simulink model "SDV_HIL"  (R2025a)
settings: Solver=VariableStepAuto  StartTime=0.0  StopTime=9999  FixedStep=0.001  RelTol=1e-3
undefined symbols (not defined in the file): Breakpoints_Fz, Cij, dspblkCoreblockFVToolHelper, eta, Fx_total_max, g, gcbh, Iz, lambda, lf, lr, mu, phi, R_eff, Tmax, xi
libraries: simulink_extras x30, slrealtimeiplib x17, slpidlib x16, simulink x10, SignalEditorBlockLib x6, dspstat3 x5, Solver_SF x3, sl3dlib x3
(part 2 of 5)

== system SDV_HIL/HIL_VCU/UDP Receive ZCU -> PC ==
  Display18 : Display
  Display26 : Display  Commented=on
  Gain1 : Gain  Gain=-1
  MATLAB Function : MATLAB Function  TreatAsAtomicUnit=on
  Median Filter : dspstat3/Median Filter  Commented=on  WindowLength=5  SimulateUsing=Interpreted execution
      settings: LibrarySourceBlock=|
      | dspfdesign/Median
      | Filter
  Mux : Mux
  Mux1 : Mux
  Rate Transition2 : RateTransition  OutPortSampleTime=0.0001
  Scope : Scope  Commented=on  NumInputPorts=2
      settings: TimeSpan=10  ActiveDisplayYMinimum=-148.76999999999998  ActiveDisplayYMaximum=138.92999999999998  DataLoggingVariableName=ScopeData62
  Scope1 : Scope  Commented=on
      settings: ActiveDisplayYMinimum=-50  ActiveDisplayYMaximum=-30  DataLoggingVariableName=ScopeData63
  Spd & Ang Convertion2 : Subsystem
  UDP Receive3 : slrealtimeiplib/UDP Receive  useHostTargetConn=off  ipAddress=10.252.62.212  localPort=4095  rcvWidth=7  rcvFmAny=on  fmAddress='10.252.62.51'  sampleTime=0.0001  enableMessage=off  maxPackets=1
  vxWheel_Ref : Outport
  AngWheel : Outport  Port=2
  wires:
  MATLAB Function/5(seqRecv) -> Display26/1
  UDP Receive3/2 -> Display18/1
  UDP Receive3/1 -> Rate Transition2/1
  Rate Transition2/1 -> MATLAB Function/1(payload)
  MATLAB Function/4(RR) -> Spd & Ang Convertion2/4(RR)
  MATLAB Function/3(RL) -> Spd & Ang Convertion2/3(RL)
  MATLAB Function/2(FR) -> Spd & Ang Convertion2/2(FR)
  MATLAB Function/1(FL) -> Spd & Ang Convertion2/1(FL)
  Spd & Ang Convertion2/1(ang_FL) -> Mux/1
  Spd & Ang Convertion2/2(ang_FR) -> Mux/2
  Spd & Ang Convertion2/3(ang_RL) -> Mux/3
  Spd & Ang Convertion2/4(ang_RR) -> Mux/4
  Mux/1 -> Gain1/1
  Spd & Ang Convertion2/5(vxWheel_FL) -> Mux1/1
  Spd & Ang Convertion2/6(vxWheel_FR) -> Mux1/2
  Spd & Ang Convertion2/7(vxWheel_RL) -> Mux1/3
  Spd & Ang Convertion2/8(vxWheel_RR) -> Mux1/4
  Median Filter/1 -> Scope/2
  Mux1/1 -> Median Filter/1, vxWheel_Ref/1, Scope/1
  Gain1/1 -> Scope1/1, AngWheel/1

== system SDV_HIL/HIL_VCU/UDP Receive Brake VCU -> PC ==
  Cast To Double : DataTypeConversion  OutDataTypeStr=double  SaturateOnIntegerOverflow=off  RndMeth=Floor
  Constant : Constant  Value=10
  Display : Display
  Display1 : Display
  Divide : Product  Inputs=*/
  MATLAB Function : MATLAB Function  TreatAsAtomicUnit=on
  Rate Transition : RateTransition  OutPortSampleTime=0.0001
  UDP Receive : slrealtimeiplib/UDP Receive  useHostTargetConn=off  ipAddress=10.252.62.212  localPort=4093  rcvWidth=4  rcvFmAny=on  fmAddress='10.10.10.10'  sampleTime=0.0001  enableMessage=off  maxPackets=1
  Brake : Outport
  wires:
  UDP Receive/2 -> Display/1
  MATLAB Function/2(seqRecv) -> Display1/1
  Constant/1 -> Divide/2
  MATLAB Function/1(Brake) -> Divide/1
  Divide/1 -> Cast To Double/1
  Cast To Double/1 -> Brake/1
  UDP Receive/1 -> Rate Transition/1
  Rate Transition/1 -> MATLAB Function/1(payload)

== system SDV_HIL/HIL_VCU/UDP Transmit PC -> VCU ==
  Vx : Inport
  Vy : Inport  Port=2
  AngWheel : Inport  Port=3
  r : Inport  Port=4
  Fy : Inport  Port=5
  Fz : Inport  Port=6
  VxWheel : Inport  Port=7
  Cast To Double : DataTypeConversion  OutDataTypeStr=double  SaturateOnIntegerOverflow=off  RndMeth=Floor
  Cast To Double1 : DataTypeConversion  OutDataTypeStr=double  SaturateOnIntegerOverflow=off  RndMeth=Floor
  Display{3..9} (7 alike) : Display
  MATLAB Function1 : MATLAB Function  TreatAsAtomicUnit=on
  UDP Send : slrealtimeiplib/UDP Send  useHostTargetConn=off  toAddress='10.252.62.129'  toPort=5100  sampleTime=0.001  enableMessage=off  ipAddress=10.252.62.212  localPort=4095
  UDP Send5 : slrealtimeiplib/UDP Send  useHostTargetConn=off  toAddress='10.252.62.55'  toPort=5055  sampleTime=0.001  enableMessage=off  ipAddress=10.252.62.212  localPort=4095
  wires:
  r/1 -> Display5/1, MATLAB Function1/4(r)
  Vy/1 -> Display3/1, MATLAB Function1/2(Vy)
  MATLAB Function1/1(payload) -> UDP Send/1, UDP Send5/1
  VxWheel/1 -> Display6/1, MATLAB Function1/7(Vx_wheel)
  AngWheel/1 -> Display4/1, MATLAB Function1/3(AngWheel)
  Fy/1 -> Display8/1, MATLAB Function1/5(Fy)
  Fz/1 -> Display9/1, MATLAB Function1/6(Fz)
  Vx/1 -> Display7/1, MATLAB Function1/1(Vx)
  MATLAB Function1/2(len) -> Cast To Double1/1, Cast To Double/1
  Cast To Double/1 -> UDP Send5/2
  Cast To Double1/1 -> UDP Send/2

== system SDV_HIL/Draft1/Sensor1/Steering System ==
  In1 : Inport
  Demux : Demux  Outputs=14
  Terminator{,1..7} (8 alike) : Terminator
  tag scope: Lat_Path=global, Lat_Targ=global, Lat_Veh=global, SteerDM=global, sideslip_L2=global, sideslip_R2=global
  wires:
  In1/1 -> Demux/1
  Demux/1 -> Terminator/1
  Demux/2 -> Terminator1/1
  Demux/3 -> Terminator2/1
  Demux/4 -> Terminator3/1
  Demux/5 -> Terminator4/1
  Demux/6 -> Terminator5/1
  Demux/7 -> [SteerDM]
  Demux/8 -> [Lat_Targ]
  Demux/9 -> [Lat_Veh]
  Demux/10 -> [Lat_Path]
  Demux/11 -> Terminator6/1
  Demux/12 -> Terminator7/1
  Demux/13 -> [sideslip_L2]
  Demux/14 -> [sideslip_R2]

== system SDV_HIL/Draft1/Sensor1/Torque Vectoring ==
  In1 : Inport
  Degrees to Radians : simulink_extras/Transformations/Degrees to Radians
  Degrees to Radians2 : simulink_extras/Transformations/Degrees to Radians
  Demux : Demux  Outputs=15
  Mux : Mux
  Mux1 : Mux
  Mux2 : Mux
  Scope{,2..5} (5 alike) : Scope  Commented=on
      Scope settings: TimeSpan=10  ActiveDisplayYMinimum=-0.018082463921750395  ActiveDisplayYMaximum=0.017846570793703453  DataLoggingVariableName=ScopeData21
      Scope2 settings: ActiveDisplayYMinimum=-1  ActiveDisplayYMaximum=1  DataLoggingVariableName=ScopeData23
      Scope3 settings: ActiveDisplayYMinimum=-106.0637202101492  ActiveDisplayYMaximum=78.0503751303972  DataLoggingVariableName=ScopeData24
      Scope4 settings: ActiveDisplayYMinimum=6542.1615610939225  ActiveDisplayYMaximum=6577.8874866083952  DataLoggingVariableName=ScopeData25
      Scope5 settings: TimeSpan=10  ActiveDisplayYMinimum=-11.664536557177181  ActiveDisplayYMaximum=101.92313834201745  DataLoggingVariableName=ScopeData61
  Scope1 : Scope  Commented=on  NumInputPorts=2
      settings: ActiveDisplayYMinimum=-15.76512014934719  ActiveDisplayYMaximum=98.336342875694754  DataLoggingVariableName=ScopeData22
  tag scope: AngWheel=global, Fy=global, Fz=global, Vx=global, Vy=global, yawrate=global
  wires:
  In1/1 -> Demux/1
  Demux/1 -> Scope5/1, [Vx]
  Demux/2 -> Scope2/1, [Vy]
  Demux/3 -> Degrees to Radians/1
  Demux/4 -> Mux2/1
  Demux/5 -> Mux2/2
  Demux/6 -> Mux2/3
  Demux/7 -> Mux2/4
  Demux/8 -> Mux1/1
  Demux/9 -> Mux1/2
  Demux/10 -> Mux1/3
  Demux/11 -> Mux1/4
  Demux/12 -> Mux/1
  Demux/13 -> Mux/2
  Demux/14 -> Mux/3
  Demux/15 -> Mux/4
  Degrees to Radians/1 -> Scope/1, [yawrate]
  Mux/1 -> Scope3/1, [Fy]
  Mux1/1 -> Scope4/1, [Fz]
  Mux2/1 -> Scope1/2, Degrees to Radians2/1
  Degrees to Radians2/1 -> Scope1/1, [AngWheel]

== system SDV_HIL/Draft1/Sensor1/Traction Control ==
  In1 : Inport
  Demux : Demux  Outputs=14
  Gain{,1..3} (4 alike) : Gain  Gain=2*pi/60
  Mux : Mux
  Mux1 : Mux
  Terminator : Terminator
  g > m/s^2 : Gain  Gain=9.80665
  tag scope: Fx=global, VxWheel=global, Vx_L1=global, Vx_L2=global, Vx_R1=global, Vx_R2=global, ax=global, w_L1=global, w_L2=global, w_R1=global, w_R2=global
  wires:
  In1/1 -> Demux/1
  Demux/2 -> [Vx_L1]
  Demux/3 -> [Vx_R1]
  Demux/4 -> [Vx_L2]
  Demux/5 -> [Vx_R2]
  Demux/1 -> Terminator/1  "Vx"
  Demux/6 -> Gain/1
  Demux/7 -> Gain1/1
  Demux/8 -> Gain2/1
  Demux/9 -> Gain3/1
  Gain/1 -> [w_L1]
  Gain1/1 -> [w_R1]
  Gain2/1 -> [w_L2]
  Gain3/1 -> [w_R2]
  Demux/10 -> g > m/s^2/1
  g > m/s^2/1 -> [ax]
  Demux/14 -> Mux/4  "Fx_R2"
  Demux/13 -> Mux/3  "Fx_L2"
  Demux/12 -> Mux/2  "Fx_R1"
  Demux/11 -> Mux/1  "Fx_L1"
  Mux/1 -> [Fx]
  [Vx_L1] -> Mux1/1
  [Vx_R1] -> Mux1/2
  [Vx_L2] -> Mux1/3
  [Vx_R2] -> Mux1/4
  Mux1/1 -> [VxWheel]

== system SDV_HIL/Draft1/Steering Input1/DLC Lateral Target  ==
  PID Controller : slpidlib/PID Controller  Controller=PID  Form=Parallel  TimeDomain=Continuous-time  UseExternalTs=off  SampleTime=-1  IntegratorMethod=Forward Euler  FilterMethod=Forward Euler  ControllerParametersSource=internal  P=12  I=0.7  UseKiTs=off  D=7  UseExternalDerivativeSource=off  N=100  UseFilter=on  TunerSelectOption=Transfer Function Based (PID Tuner App)  InitialConditionSource=internal  InitialConditionForIntegrator=0  InitialConditionForFilter=0  DifferentiatorICPrevScaledInput=0  ExternalReset=none  TrackingMode=off  Kt=1  LimitOutput=off  SatLimitsSource=internal  UpperSaturationLimit=inf  LowerSaturationLimit=-inf  LinearizeAsGain=on  AntiWindupMode=none  Kb=1  LimitIntegrator=off  UpperIntegratorSaturationLimit=inf  LowerIntegratorSaturationLimit=-inf  POutMin=[]  POutMax=[]  IOutMin=[]  IOutMax=[]  DOutMin=[]  DOutMax=[]  NOutMin=[]  NOutMax=[]  SumOutMin=[]  SumOutMax=[]  SaturationOutMin=[]  SaturationOutMax=[]  PParamMin=[]  PParamMax=[]  IParamMin=[]  IParamMax=[]  DParamMin=[]  DParamMax=[]  NParamMin=[]  NParamMax=[]  KbParamMin=[]  KbParamMax=[]  KtParamMin=[]  KtParamMax=[]  KbOutMin=[]  KbOutMax=[]  KtOutMin=[]  KtOutMax=[]  IntegratorOutMin=[]  IntegratorOutMax=[]  FilterOutMin=[]  FilterOutMax=[]  SumI1OutMin=[]  SumI1OutMax=[]  SumI2OutMin=[]  SumI2OutMax=[]  SumI3OutMin=[]  SumI3OutMax=[]  SumI4OutMin=[]  SumI4OutMax=[]  SumDOutMin=[]  SumDOutMax=[]  DifferentiatorOutMin=[]  DifferentiatorOutMax=[]  FilterDiffOutCoefMin=[]  FilterDiffOutCoefMax=[]  ReciprocalOutMin=[]  ReciprocalOutMax=[]  SumDenOutMin=[]  SumDenOutMax=[]  SumNumOutMin=[]  SumNumOutMax=[]  DivideOutMin=[]  DivideOutMax=[]  UdiffTsProdOutMin=[]  UdiffTsProdOutMax=[]  NTsProdOutMin=[]  NTsProdOutMax=[]  UintegralTsProdOutMin=[]  UintegralTsProdOutMax=[]  UngainTsProdOutMin=[]  UngainTsProdOutMax=[]  ClampingZeroOutDataTypeStr=Inherit: Inherit via back propagation  ClampingZeroOutMin=[]  ClampingZeroOutMax=[]  FilterDenConstantOutDataTypeStr=Inherit: Inherit via back propagation  FilterDenConstantOutMin=[]  FilterDenConstantOutMax=[]  PCopyOutDataTypeStr=Inherit: Inherit via back propagation  PCopyOutMin=[]  PCopyOutMax=[]  NCopyOutDataTypeStr=Inherit: Inherit via back propagation  NCopyOutMin=[]  NCopyOutMax=[]  IntegratorContinuousStateAttributes=''  IntegratorStateMustResolveToSignalObject=off  IntegratorRTWStateStorageClass=Auto  FilterContinuousStateAttributes=''  FilterStateMustResolveToSignalObject=off  FilterRTWStateStorageClass=Auto  ParallelPVariant=InternalParameters  IdealPVariant=Disabled  IVariant=InternalParameters  DVariant=InternalParameters  IntegratorVariant=Continuous  SatVariant=Disabled  AWVariant=Passthrough  PCopyVariant=Disabled  TRVariant=Disabled  FdbkBlocksVariant=Forward  IdealPFdbkVariant=Disabled  SatFdbkVariant=Disabled  DerivativeFilterVariant=ContFilter  NVariant=InternalParameters  NCopyVariant=Disabled  FilterICVariant=InternalICsFilter  IntegratorICVariant=InternalICs  ExternalResetVariant=Disabled  TRSumVariant=Passthrough  SumFdbkVariant=Disabled  SumVariant=Sum_PID  TsampFilterVariant=InternalTs  TsampNgainVariant=Passthrough  TsampIntegralVariant=Disabled_SignalSpec  ExternalSaturationOutDataTypeStr=Inherit: Same as second input  DerivativeSourceVariant=ErrorSignal  PreIntVariant=InternalPreInt
  Saturation : Saturate  UpperLimit=40  LowerLimit=-40
  Scope1 : Scope
      settings: ActiveDisplayYMinimum=-50  ActiveDisplayYMaximum=50  DataLoggingVariableName=ScopeData17
  Scope2 : Scope
      settings: ActiveDisplayYMinimum=-26.333159271082913  ActiveDisplayYMaximum=27.304615856489622  DataLoggingVariableName=ScopeData18
  Sum : Sum  Inputs=|+-
  Out1 : Outport
  wires:
  [Lat_Veh] -> Sum/2
  [Lat_Targ] -> Sum/1
  Sum/1 -> Scope2/1, PID Controller/1
  PID Controller/1 -> Saturation/1
  Saturation/1 -> Out1/1, Scope1/1

== system SDV_HIL/Draft1/Steering Input1/DLC SteerDM ==
  1-D Lookup Table : Lookup_n-D  NumberOfTableDimensions=1  BreakpointsForDimension1=[-540 0 540]  Table=[-40 0 40]  InternalRulePriority=Speed  RndMeth=Simplest
  Saturation : Saturate  UpperLimit=40  LowerLimit=-40
  Scope1 : Scope  NumInputPorts=3
      settings: ActiveDisplayYMinimum=-1  ActiveDisplayYMaximum=1  DataLoggingVariableName=ScopeData19
  Str : Outport
  wires:
  Saturation/1 -> Str/1, Scope1/1
  1-D Lookup Table/1 -> Scope1/2, Saturation/1
  [SteerDM] -> 1-D Lookup Table/1, Scope1/3

== system SDV_HIL/Draft1/Steering Input1/Driver Logi G29 ==
  Add : Sum
  Add1 : Sum
  Constant : Constant  Value=50
  Constant1 : Constant  Value=6
  Demux : Demux
  Display{,1..2,4..6} (6 alike) : Display
  Gain3 : Gain  Gain=-6
  Gain4 : Gain  Gain=-50
  Gain5 : Gain  Gain=40
  Goto2 : Goto  Commented=on  GotoTag=Brake_pedal  TagVisibility=global
  MATLAB Function : MATLAB Function  TreatAsAtomicUnit=on
  Selector : Selector  InputPortWidth=25  IndexOptions=Index vector (dialog)  Indices=[1]  OutputSizes=1
  Simulation 3D Joystick : sl3dlib/Simulation 3D/Hardware Interface/Simulation 3D Joystick  joyid=1  adjustports=on  forcefeed=off
  Switch : Switch  Criteria=u2 > Threshold  SaturateOnIntegerOverflow=off  InputSameDT=off
  Switch1 : Switch  Criteria=u2 > Threshold  SaturateOnIntegerOverflow=off  InputSameDT=off
  Terminator : Terminator
  Terminator2 : Terminator
  Zero : Constant  Value=0  OutDataTypeStr=Inherit: Inherit via back propagation
  Zero1 : Constant  Value=0  OutDataTypeStr=Inherit: Inherit via back propagation
  tag scope: Steer=global, Throttle=global
  wires:
  Simulation 3D Joystick/3 -> Terminator/1
  Zero1/1 -> Switch1/3
  Switch1/1 -> Display5/1, [Throttle]
  Add/1 -> Switch1/1
  Zero/1 -> Switch/3
  MATLAB Function/1(state) -> Display4/1, Switch/2, Switch1/2
  Selector/1 -> MATLAB Function/1(btn)
  Gain5/1 -> [Steer], Display2/1
  Add1/1 -> Display6/1, Goto2/1
  Constant1/1 -> Add1/2
  Gain3/1 -> Add1/1
  Demux/3 -> Gain3/1
  Demux/2 -> Gain4/1
  Demux/1 -> Gain5/1
  Demux/4 -> Terminator2/1
  Simulation 3D Joystick/1 -> Display/1, Demux/1, Switch/1
  Gain4/1 -> Add/1
  Constant/1 -> Add/2
  Simulation 3D Joystick/2 -> Selector/1, Display1/1

== system SDV_HIL/Draft1/Steering Input1/Sine with Dwell ==
  Gain : Gain  Gain=5
  Sine with Dwell : SignalEditorBlockLib/Signal Editor  FileName=Sine with Dwell.mat  ActiveScenario=Scenario  ActiveSignal=Signal 1  IsBus=off  OutputBusObjectStr=Bus: BusObject  SampleTime=0  ZeroCross=off  OutputAfterFinalValue=Setting to zero  Unit=inherit  PreserveSignalName=on  ApplySigPropsToAllScenarios=on  ApplySigPropsToAllSignals=off  SignalPropertySource=Dialog parameters
  Str : Outport
  wires:
  Sine with Dwell/1 -> Gain/1
  Gain/1 -> Str/1

== system SDV_HIL/Draft1/Steering Input1/Sine with Dwell shifted ==
  Gain : Gain  Gain=5
  Sine with Dwell : SignalEditorBlockLib/Signal Editor  FileName=SineWithDwell_shifted.mat  ActiveScenario=Scenario  ActiveSignal=Signal 1  IsBus=off  OutputBusObjectStr=Bus: BusObject  SampleTime=0  ZeroCross=off  OutputAfterFinalValue=Setting to zero  Unit=inherit  PreserveSignalName=on  ApplySigPropsToAllScenarios=on  ApplySigPropsToAllSignals=off  SignalPropertySource=Dialog parameters
  Str : Outport
  wires:
  Gain/1 -> Str/1
  Sine with Dwell/1 -> Gain/1

== system SDV_HIL/Draft1/Steering Input1/Subsystem ==
  In1 : Inport
  Str : Outport
  wires:
  In1/1 -> Str/1

== system SDV_HIL/Draft1/Subsystem1/Motor1 ==
  SpdTCS : Inport
  Demux : Demux
  Gain : Gain  Gain=4
  Mux : Mux
  PID Controller : slpidlib/PID Controller  Controller=PID  Form=Parallel  TimeDomain=Continuous-time  UseExternalTs=off  SampleTime=-1  IntegratorMethod=Forward Euler  FilterMethod=Forward Euler  ControllerParametersSource=internal  P=20  I=0.05  UseKiTs=off  D=1  UseExternalDerivativeSource=off  N=100  UseFilter=on  TunerSelectOption=Transfer Function Based (PID Tuner App)  InitialConditionSource=internal  InitialConditionForIntegrator=0  InitialConditionForFilter=0  DifferentiatorICPrevScaledInput=0  ExternalReset=none  TrackingMode=off  Kt=1  LimitOutput=off  SatLimitsSource=internal  UpperSaturationLimit=inf  LowerSaturationLimit=-inf  LinearizeAsGain=on  AntiWindupMode=none  Kb=1  LimitIntegrator=off  UpperIntegratorSaturationLimit=inf  LowerIntegratorSaturationLimit=-inf  POutMin=[]  POutMax=[]  IOutMin=[]  IOutMax=[]  DOutMin=[]  DOutMax=[]  NOutMin=[]  NOutMax=[]  SumOutMin=[]  SumOutMax=[]  SaturationOutMin=[]  SaturationOutMax=[]  PParamMin=[]  PParamMax=[]  IParamMin=[]  IParamMax=[]  DParamMin=[]  DParamMax=[]  NParamMin=[]  NParamMax=[]  KbParamMin=[]  KbParamMax=[]  KtParamMin=[]  KtParamMax=[]  KbOutMin=[]  KbOutMax=[]  KtOutMin=[]  KtOutMax=[]  IntegratorOutMin=[]  IntegratorOutMax=[]  FilterOutMin=[]  FilterOutMax=[]  SumI1OutMin=[]  SumI1OutMax=[]  SumI2OutMin=[]  SumI2OutMax=[]  SumI3OutMin=[]  SumI3OutMax=[]  SumI4OutMin=[]  SumI4OutMax=[]  SumDOutMin=[]  SumDOutMax=[]  DifferentiatorOutMin=[]  DifferentiatorOutMax=[]  FilterDiffOutCoefMin=[]  FilterDiffOutCoefMax=[]  ReciprocalOutMin=[]  ReciprocalOutMax=[]  SumDenOutMin=[]  SumDenOutMax=[]  SumNumOutMin=[]  SumNumOutMax=[]  DivideOutMin=[]  DivideOutMax=[]  UdiffTsProdOutMin=[]  UdiffTsProdOutMax=[]  NTsProdOutMin=[]  NTsProdOutMax=[]  UintegralTsProdOutMin=[]  UintegralTsProdOutMax=[]  UngainTsProdOutMin=[]  UngainTsProdOutMax=[]  ClampingZeroOutDataTypeStr=Inherit: Inherit via back propagation  ClampingZeroOutMin=[]  ClampingZeroOutMax=[]  FilterDenConstantOutDataTypeStr=Inherit: Inherit via back propagation  FilterDenConstantOutMin=[]  FilterDenConstantOutMax=[]  PCopyOutDataTypeStr=Inherit: Inherit via back propagation  PCopyOutMin=[]  PCopyOutMax=[]  NCopyOutDataTypeStr=Inherit: Inherit via back propagation  NCopyOutMin=[]  NCopyOutMax=[]  IntegratorContinuousStateAttributes=''  IntegratorStateMustResolveToSignalObject=off  IntegratorRTWStateStorageClass=Auto  FilterContinuousStateAttributes=''  FilterStateMustResolveToSignalObject=off  FilterRTWStateStorageClass=Auto  ParallelPVariant=InternalParameters  IdealPVariant=Disabled  IVariant=InternalParameters  DVariant=InternalParameters  IntegratorVariant=Continuous  SatVariant=Disabled  AWVariant=Passthrough  PCopyVariant=Disabled  TRVariant=Disabled  FdbkBlocksVariant=Forward  IdealPFdbkVariant=Disabled  SatFdbkVariant=Disabled  DerivativeFilterVariant=ContFilter  NVariant=InternalParameters  NCopyVariant=Disabled  FilterICVariant=InternalICsFilter  IntegratorICVariant=InternalICs  ExternalResetVariant=Disabled  TRSumVariant=Passthrough  SumFdbkVariant=Disabled  SumVariant=Sum_PID  TsampFilterVariant=InternalTs  TsampNgainVariant=Passthrough  TsampIntegralVariant=Disabled_SignalSpec  ExternalSaturationOutDataTypeStr=Inherit: Same as second input  DerivativeSourceVariant=ErrorSignal  PreIntVariant=InternalPreInt
  Saturation : Saturate  UpperLimit=256  LowerLimit=-256
  Scope : Scope  NumInputPorts=2
      settings: ActiveDisplayYMinimum=-100.56314203320845  ActiveDisplayYMaximum=848.44383025663615  DataLoggingVariableName=ScopeData8
  Scope1 : Scope
      settings: ActiveDisplayYMinimum=-320  ActiveDisplayYMaximum=320  DataLoggingVariableName=ScopeData15
  Scope2 : Scope
      settings: ActiveDisplayYMinimum=-15.146247733878647  ActiveDisplayYMaximum=78.344930970085713  DataLoggingVariableName=ScopeData34
  Subsystem : Subsystem
  Subsystem1 : Subsystem
  Subsystem2 : Subsystem
  Subsystem3 : Subsystem
  Sum{,1..3} (4 alike) : Sum  Inputs=|+-
  Traction Control : Subsystem
  Out1 : Outport
  wires:
  Subsystem3/1(Out1) -> Sum3/1
  Subsystem2/1(Out1) -> Sum2/1
  Subsystem1/1(Out1) -> Sum1/1
  Subsystem/1(Out1) -> Sum/1
  SpdTCS/1 -> Traction Control/1(SpdTCS)
  Traction Control/1(Out1) -> Demux/1
  Saturation/1 -> Scope1/1, Gain/1
  Gain/1 -> Out1/1
  PID Controller/1 -> Saturation/1
  Mux/1 -> PID Controller/1, Scope2/1
  Sum/1 -> Mux/1
  [Vx_R2] -> Sum3/2
  Sum3/1 -> Mux/4
  [Vx_L2] -> Sum2/2
  Sum2/1 -> Mux/3
  Sum1/1 -> Mux/2
  [Vx_R1] -> Sum1/2
  [Vx_L1] -> Sum/2, Scope/2
  Demux/4 -> Subsystem3/1(In1)
  Demux/3 -> Subsystem2/1(In1)
  Demux/2 -> Subsystem1/1(In1)
  Demux/1 -> Subsystem/1(In1)

== system SDV_HIL/Draft1/Subsystem1/Steering1 ==
  Ang_reff : Inport
  Mzd : Inport  Port=2
  "Cr, calculation" : Subsystem
      settings: PortSchema="{\"entries\":[{\"content\":{\"sides\":[{\"content\":{},\"type\":\"ConnectorPlacement.EquallySpacedRectSide\",\"uuid\":\"05ba1d87-4e1a-4b14-8204-c87cb45244d4\"},{\"content\":{\"connectorIds\":[\"In1\"],\"side\":\"RIGHT\"},\"type\":\"ConnectorPlacement.EquallySpacedRectSide\",\"uuid\":\"db79dace-63f7-4aff-a5f3-b83b2cb69b1b\"},{\"content\":{\"side\":\"TOP\"},\"type\":\"ConnectorPlacement.EquallySpacedRectSide\",\"uuid\":\"14afade6-4b72-407c-9595-a03dfacfb377\"}]},\"type\":\"ConnectorPlacement.EquallySpacedConnector\",\"uuid\":\"7a804c5d-435f-4613-b38b-74b890646bdf\"}],\"packageUris\":[\"http://schema.mathworks.com/mf0/Connector/R2020b\"],\"version\":\"1.0\"}"
  Dynamic : Subsystem
  Scope : Scope
      settings: ActiveDisplayYMinimum=-10.213571223777571  ActiveDisplayYMaximum=10.459894996843868  DataLoggingVariableName=ScopeData52
  Scope1 : Scope
      settings: ActiveDisplayYMinimum=-5.9590075157814937  ActiveDisplayYMaximum=5.69631275538866  DataLoggingVariableName=ScopeData57
  Deg : Outport
  wires:
  Mzd/1 -> Dynamic/2(Mz)
  Ang_reff/1 -> Dynamic/1(In2), Scope1/1
  Dynamic/1(Deg) -> Scope/1, "Cr, calculation"/1(In1), Deg/1

== system SDV_HIL/Draft1/Subsystem1/Torque to Speed Distribution1 ==
  note: Vx_ref = Vx(1+gain*pi)
  TqWheel : Inport
  Spd : Inport  Port=2
  Add : Sum
  Add1 : Sum
  Constant : Constant
  Demux : Demux
  Gain : Gain  Gain=1/256
  PID Controller : slpidlib/PID Controller  Controller=PID  Form=Parallel  TimeDomain=Continuous-time  UseExternalTs=off  SampleTime=-1  IntegratorMethod=Forward Euler  FilterMethod=Forward Euler  ControllerParametersSource=internal  P=12  I=0.4  UseKiTs=off  D=0  UseExternalDerivativeSource=off  N=100  UseFilter=on  TunerSelectOption=Transfer Function Based (PID Tuner App)  InitialConditionSource=internal  InitialConditionForIntegrator=0  InitialConditionForFilter=0  DifferentiatorICPrevScaledInput=0  ExternalReset=none  TrackingMode=off  Kt=1  LimitOutput=off  SatLimitsSource=internal  UpperSaturationLimit=inf  LowerSaturationLimit=-inf  LinearizeAsGain=on  AntiWindupMode=none  Kb=1  LimitIntegrator=off  UpperIntegratorSaturationLimit=inf  LowerIntegratorSaturationLimit=-inf  POutMin=[]  POutMax=[]  IOutMin=[]  IOutMax=[]  DOutMin=[]  DOutMax=[]  NOutMin=[]  NOutMax=[]  SumOutMin=[]  SumOutMax=[]  SaturationOutMin=[]  SaturationOutMax=[]  PParamMin=[]  PParamMax=[]  IParamMin=[]  IParamMax=[]  DParamMin=[]  DParamMax=[]  NParamMin=[]  NParamMax=[]  KbParamMin=[]  KbParamMax=[]  KtParamMin=[]  KtParamMax=[]  KbOutMin=[]  KbOutMax=[]  KtOutMin=[]  KtOutMax=[]  IntegratorOutMin=[]  IntegratorOutMax=[]  FilterOutMin=[]  FilterOutMax=[]  SumI1OutMin=[]  SumI1OutMax=[]  SumI2OutMin=[]  SumI2OutMax=[]  SumI3OutMin=[]  SumI3OutMax=[]  SumI4OutMin=[]  SumI4OutMax=[]  SumDOutMin=[]  SumDOutMax=[]  DifferentiatorOutMin=[]  DifferentiatorOutMax=[]  FilterDiffOutCoefMin=[]  FilterDiffOutCoefMax=[]  ReciprocalOutMin=[]  ReciprocalOutMax=[]  SumDenOutMin=[]  SumDenOutMax=[]  SumNumOutMin=[]  SumNumOutMax=[]  DivideOutMin=[]  DivideOutMax=[]  UdiffTsProdOutMin=[]  UdiffTsProdOutMax=[]  NTsProdOutMin=[]  NTsProdOutMax=[]  UintegralTsProdOutMin=[]  UintegralTsProdOutMax=[]  UngainTsProdOutMin=[]  UngainTsProdOutMax=[]  ClampingZeroOutDataTypeStr=Inherit: Inherit via back propagation  ClampingZeroOutMin=[]  ClampingZeroOutMax=[]  FilterDenConstantOutDataTypeStr=Inherit: Inherit via back propagation  FilterDenConstantOutMin=[]  FilterDenConstantOutMax=[]  PCopyOutDataTypeStr=Inherit: Inherit via back propagation  PCopyOutMin=[]  PCopyOutMax=[]  NCopyOutDataTypeStr=Inherit: Inherit via back propagation  NCopyOutMin=[]  NCopyOutMax=[]  IntegratorContinuousStateAttributes=''  IntegratorStateMustResolveToSignalObject=off  IntegratorRTWStateStorageClass=Auto  FilterContinuousStateAttributes=''  FilterStateMustResolveToSignalObject=off  FilterRTWStateStorageClass=Auto  ParallelPVariant=InternalParameters  IdealPVariant=Disabled  IVariant=InternalParameters  DVariant=InternalParameters  IntegratorVariant=Continuous  SatVariant=Disabled  AWVariant=Passthrough  PCopyVariant=Disabled  TRVariant=Disabled  FdbkBlocksVariant=Forward  IdealPFdbkVariant=Disabled  SatFdbkVariant=Disabled  DerivativeFilterVariant=ContFilter  NVariant=InternalParameters  NCopyVariant=Disabled  FilterICVariant=InternalICsFilter  IntegratorICVariant=InternalICs  ExternalResetVariant=Disabled  TRSumVariant=Passthrough  SumFdbkVariant=Disabled  SumVariant=Sum_PID  TsampFilterVariant=InternalTs  TsampNgainVariant=Passthrough  TsampIntegralVariant=Disabled_SignalSpec  ExternalSaturationOutDataTypeStr=Inherit: Same as second input  DerivativeSourceVariant=ErrorSignal  PreIntVariant=InternalPreInt
  Product : Product
  Saturation : Saturate  UpperLimit=inf  LowerLimit=-5
  Saturation1 : Saturate  UpperLimit=100  LowerLimit=-100
  Scope : Scope  NumInputPorts=4
      settings: ActiveDisplayYMinimum=90.162639673500763  ActiveDisplayYMaximum=110.8541393507157  DataLoggingVariableName=ScopeData3
  Scope1 : Scope
      settings: ActiveDisplayYMinimum=-1  ActiveDisplayYMaximum=1  DataLoggingVariableName=ScopeData11
  Scope2 : Scope  NumInputPorts=2
      settings: ActiveDisplayYMinimum=99.866338620486374  ActiveDisplayYMaximum=100.03544324263167  DataLoggingVariableName=ScopeData14
  Scope3 : Scope
      settings: ActiveDisplayYMinimum=-0.035443242631677307  ActiveDisplayYMaximum=0.13366137951363122  DataLoggingVariableName=ScopeData31
  Scope4 : Scope
      settings: ActiveDisplayYMinimum=0.907762016097617  ActiveDisplayYMaximum=1.1071006385683808  DataLoggingVariableName=ScopeData33
  Sum : Sum  Inputs=|+-
  Tuning : Gain  Gain=0.08
  SpdWheel : Outport
  wires:
  [initialCondition] -> Add1/2
  Add1/1 -> Product/1, Scope1/1
  Saturation1/1 -> Add1/1
  PID Controller/1 -> Saturation1/1
  Saturation/1 -> Scope3/1, PID Controller/1
  Sum/1 -> Saturation/1
  [Vx] -> Sum/2, Scope2/2
  Spd/1 -> Sum/1, Scope2/1
  Demux/4 -> Scope/4
  Demux/3 -> Scope/3
  Demux/2 -> Scope/2
  Demux/1 -> Scope/1
  Product/1 -> SpdWheel/1, Demux/1
  Add/1 -> Product/2, Scope4/1
  Constant/1 -> Add/2
  Tuning/1 -> Add/1
  Gain/1 -> Tuning/1
  TqWheel/1 -> Gain/1

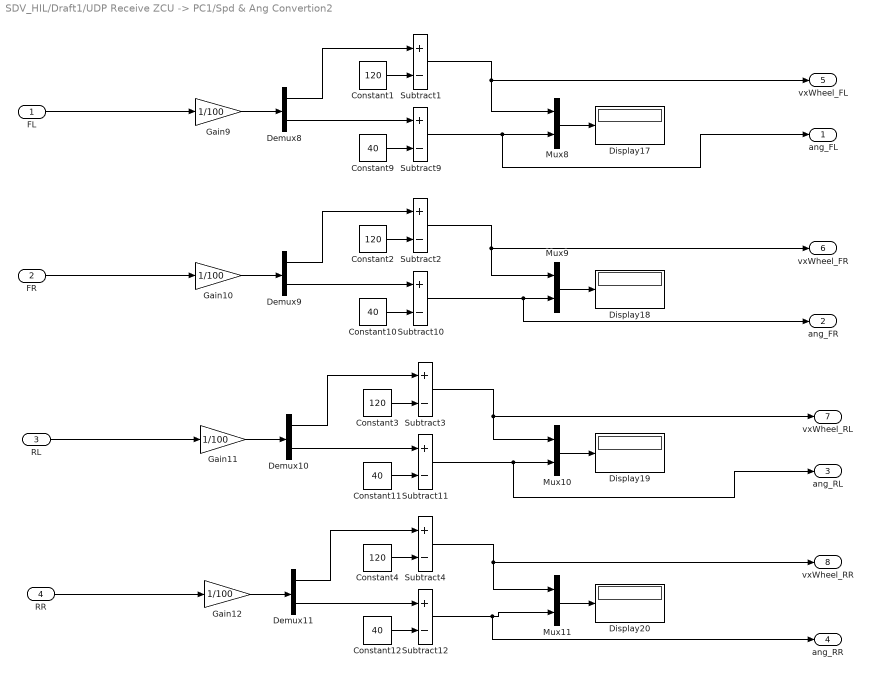
== system SDV_HIL/Draft1/UDP Receive ZCU -> PC1/Spd & Ang Convertion2 ==
  FL : Inport
  FR : Inport  Port=2
  RL : Inport  Port=3
  RR : Inport  Port=4
  Constant{1..4} (4 alike) : Constant  Value=120
  Constant{9..12} (4 alike) : Constant  Value=40
  Demux{8..11} (4 alike) : Demux  Outputs=2
  Display{17..20} (4 alike) : Display
  Gain{9..12} (4 alike) : Gain  Gain=1/100
  Mux{8..11} (4 alike) : Mux  Inputs=2
  Subtract{1..4,9..12} (8 alike) : Sum  Inputs=+-
  ang_FL : Outport
  ang_FR : Outport  Port=2
  ang_RL : Outport  Port=3
  ang_RR : Outport  Port=4
  vxWheel_FL : Outport  Port=5
  vxWheel_FR : Outport  Port=6
  vxWheel_RL : Outport  Port=7
  vxWheel_RR : Outport  Port=8
  wires:
  Gain12/1 -> Demux11/1
  Gain9/1 -> Demux8/1
  RR/1 -> Gain12/1
  FR/1 -> Gain10/1
  Gain10/1 -> Demux9/1
  Constant10/1 -> Subtract10/2
  Mux9/1 -> Display18/1
  Mux8/1 -> Display17/1
  FL/1 -> Gain9/1
  Mux10/1 -> Display19/1
  Constant12/1 -> Subtract12/2
  Mux11/1 -> Display20/1
  Gain11/1 -> Demux10/1
  Constant11/1 -> Subtract11/2
  Constant9/1 -> Subtract9/2
  RL/1 -> Gain11/1
  Subtract9/1 -> ang_FL/1, Mux8/2
  Subtract10/1 -> ang_FR/1, Mux9/2
  Subtract11/1 -> ang_RL/1, Mux10/2
  Subtract12/1 -> ang_RR/1, Mux11/2
  Constant1/1 -> Subtract1/2
  Demux8/1 -> Subtract1/1
  Subtract1/1 -> vxWheel_FL/1, Mux8/1
  Constant2/1 -> Subtract2/2
  Demux9/1 -> Subtract2/1
  Subtract2/1 -> vxWheel_FR/1, Mux9/1
  Constant3/1 -> Subtract3/2
  Demux10/1 -> Subtract3/1
  Subtract3/1 -> vxWheel_RL/1, Mux10/1
  Constant4/1 -> Subtract4/2
  Demux11/1 -> Subtract4/1
  Subtract4/1 -> vxWheel_RR/1, Mux11/1
  Demux8/2 -> Subtract9/1
  Demux9/2 -> Subtract10/1
  Demux10/2 -> Subtract11/1
  Demux11/2 -> Subtract12/1

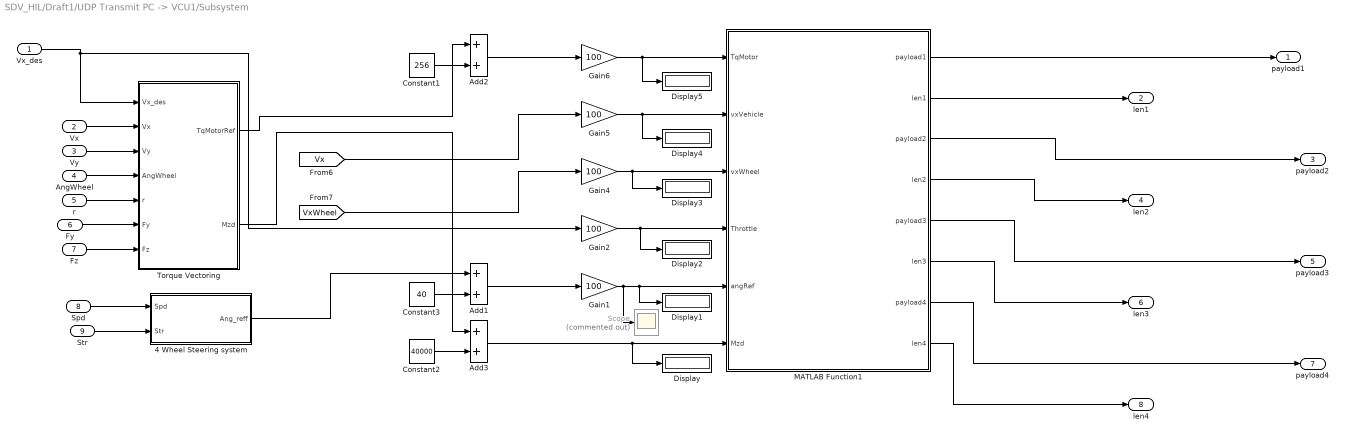
== system SDV_HIL/Draft1/UDP Transmit PC -> VCU1/Subsystem ==
  Vx_des : Inport
  Vx : Inport  Port=2
  Vy : Inport  Port=3
  AngWheel : Inport  Port=4
  r : Inport  Port=5
  Fy : Inport  Port=6
  Fz : Inport  Port=7
  Spd : Inport  Port=8
  Str : Inport  Port=9
  4 Wheel Steering system : Subsystem
  Add1 : Sum
  Add2 : Sum
  Add3 : Sum
  Constant1 : Constant  Value=256
  Constant2 : Constant  Value=40000
  Constant3 : Constant  Value=40
  Display{,1..5} (6 alike) : Display
  Gain{1..2,4..6} (5 alike) : Gain  Gain=100
  MATLAB Function1 : MATLAB Function  TreatAsAtomicUnit=on
  Scope : Scope  Commented=on
      settings: ActiveDisplayYMinimum=2651  ActiveDisplayYMaximum=5349  DataLoggingVariableName=ScopeData60
  Torque Vectoring : Subsystem
  payload1 : Outport
  len1 : Outport  Port=2
  payload2 : Outport  Port=3
  len2 : Outport  Port=4
  payload3 : Outport  Port=5
  len3 : Outport  Port=6
  payload4 : Outport  Port=7
  len4 : Outport  Port=8
  wires:
  Gain6/1 -> Display5/1, MATLAB Function1/1(TqMotor)
  Constant2/1 -> Add3/2
  Gain1/1 -> Display1/1, MATLAB Function1/5(angRef), Scope/1
  Gain2/1 -> Display2/1, MATLAB Function1/4(Throttle)
  AngWheel/1 -> Torque Vectoring/4(AngWheel)
  Fz/1 -> Torque Vectoring/7(Fz)
  4 Wheel Steering system/1(Ang_reff) -> Add1/1
  Vx_des/1 -> Torque Vectoring/1(Vx_des), Gain2/1
  Str/1 -> 4 Wheel Steering system/2(Str)
  MATLAB Function1/6(len3) -> len3/1
  r/1 -> Torque Vectoring/5(r)
  Gain5/1 -> Display4/1, MATLAB Function1/2(vxVehicle)
  Add3/1 -> Display/1, MATLAB Function1/6(Mzd)
  Torque Vectoring/1(TqMotorRef) -> Add2/1
  Torque Vectoring/2(Mzd) -> Add3/1
  Constant3/1 -> Add1/2
  Add2/1 -> Gain6/1
  Vy/1 -> Torque Vectoring/3(Vy)
  MATLAB Function1/3(payload2) -> payload2/1
  [VxWheel] -> Gain4/1
  Constant1/1 -> Add2/2
  Gain4/1 -> Display3/1, MATLAB Function1/3(vxWheel)
  Add1/1 -> Gain1/1
  MATLAB Function1/1(payload1) -> payload1/1
  MATLAB Function1/8(len4) -> len4/1
  [Vx] -> Gain5/1
  Vx/1 -> Torque Vectoring/2(Vx)
  Spd/1 -> 4 Wheel Steering system/1(Spd)
  MATLAB Function1/4(len2) -> len2/1
  Fy/1 -> Torque Vectoring/6(Fy)
  MATLAB Function1/7(payload4) -> payload4/1
  MATLAB Function1/5(payload3) -> payload3/1
  MATLAB Function1/2(len1) -> len1/1

== system SDV_HIL/Draft1/VCU Com1/UDP Receive <- VCU1 ==
  Constant1 : Constant  Value=40
  Display{,1..2,18,25..26} (6 alike) : Display
  Gain2 : Gain  Gain=1/100
  Gain3 : Gain  Gain=1/100
  Gain4 : Gain  Gain=12/100
  MATLAB Function : MATLAB Function  TreatAsAtomicUnit=on
  Rate Transition2 : RateTransition  OutPortSampleTime=0.0001
  Spd & Ang Convertion2 : Subsystem
  Subtract1 : Sum  Inputs=+-
  UDP Receive3 : slrealtimeiplib/UDP Receive  useHostTargetConn=off  ipAddress=10.252.62.212  localPort=4093  rcvWidth=19  rcvFmAny=off  fmAddress='10.252.62.111'  sampleTime=-1  enableMessage=off  maxPackets=1
  tag scope: BrakeRef=global, SteerDM=global, Throttle=global, angCacl_FL=global, angCacl_FR=global, angCacl_RL=global, angCacl_RR=global, seqCalc=global, seqRef=global, spdCalc_FL=global, spdCalc_FR=global, spdCalc_RL=global, spdCalc_RR=global
  wires:
  MATLAB Function/9(seqCalc) -> [seqCalc], Display26/1
  MATLAB Function/8(seqRef) -> [seqRef], Display25/1
  MATLAB Function/3(Brake) -> Gain4/1
  Gain4/1 -> Display2/1, [BrakeRef]
  MATLAB Function/2(Throttle) -> Gain3/1
  MATLAB Function/1(Steer) -> Gain2/1
  Gain2/1 -> Subtract1/1
  Constant1/1 -> Subtract1/2
  UDP Receive3/2 -> Display18/1
  UDP Receive3/1 -> Rate Transition2/1
  Rate Transition2/1 -> MATLAB Function/1(payload)
  MATLAB Function/7(RR) -> Spd & Ang Convertion2/4(RR)
  MATLAB Function/6(RL) -> Spd & Ang Convertion2/3(RL)
  MATLAB Function/5(FR) -> Spd & Ang Convertion2/2(FR)
  MATLAB Function/4(FL) -> Spd & Ang Convertion2/1(FL)
  Spd & Ang Convertion2/4(ang_RR) -> [angCacl_RR]
  Spd & Ang Convertion2/7(spd_RL) -> [spdCalc_RL]
  Spd & Ang Convertion2/6(spd_FR) -> [spdCalc_FR]
  Spd & Ang Convertion2/2(ang_FR) -> [angCacl_FR]
  Spd & Ang Convertion2/5(spd_FL) -> [spdCalc_FL]
  Spd & Ang Convertion2/1(ang_FL) -> [angCacl_FL]
  Spd & Ang Convertion2/3(ang_RL) -> [angCacl_RL]
  Spd & Ang Convertion2/8(spd_RR) -> [spdCalc_RR]
  Gain3/1 -> Display1/1, [Throttle]
  Subtract1/1 -> Display/1, [SteerDM]

== system SDV_HIL/Draft1/VCU Com1/UDP Send -> VCU1 ==
  Add1 : Sum
  Constant3 : Constant  Value=40
  Data Type Conversion : DataTypeConversion  OutDataTypeStr=double  SaturateOnIntegerOverflow=off  RndMeth=Floor
  Data Type Conversion1 : DataTypeConversion  OutDataTypeStr=double  SaturateOnIntegerOverflow=off  RndMeth=Floor
  Display{,1..2,4} (4 alike) : Display
  Gain1 : Gain  Gain=100
  Gain4 : Gain  Gain=100
  Gain5 : Gain  Gain=100
  MATLAB Function1 : MATLAB Function  TreatAsAtomicUnit=on
  Rate Transition1 : RateTransition  OutPortSampleTime=0.001
  Saturation : Saturate  UpperLimit=100  LowerLimit=0
  Scope : Scope
      settings: ActiveDisplayYMinimum=-25.749999999999993  ActiveDisplayYMaximum=231.75  DataLoggingVariableName=ScopeData31
  UDP Send1 : slrealtimeiplib/UDP Send  useHostTargetConn=off  toAddress='10.252.62.111'  toPort=5055  sampleTime=0.001  enableMessage=off  ipAddress=10.252.62.212  localPort=4093
  UDP Send2 : slrealtimeiplib/UDP Send  useHostTargetConn=off  toAddress='10.252.62.111'  toPort=5055  sampleTime=0.001  enableMessage=off  ipAddress=10.252.62.212  localPort=4093
  wires:
  MATLAB Function1/4(len2) -> Data Type Conversion1/1
  MATLAB Function1/3(payload2) -> Rate Transition1/1
  Rate Transition1/1 -> Display2/1, Scope/1, UDP Send2/1
  Data Type Conversion1/1 -> UDP Send2/2, Display1/1
  MATLAB Function1/2(len1) -> Data Type Conversion/1
  Gain5/1 -> MATLAB Function1/3(vxVehicle)
  Gain1/1 -> MATLAB Function1/1(angWheel)
  Gain4/1 -> MATLAB Function1/2(spdWheel)
  Data Type Conversion/1 -> UDP Send1/2, Display/1
  [Vx_Wheel] -> Gain4/1
  [AngWheel] -> Add1/1
  [Vx] -> Saturation/1
  MATLAB Function1/1(payload1) -> Display4/1, UDP Send1/1
  Constant3/1 -> Add1/2
  Add1/1 -> Gain1/1
  [seqCalc] -> MATLAB Function1/4(seqCalc)
  Saturation/1 -> Gain5/1

== system SDV_HIL/HIL/Driver/DLC SteerDM ==
  1-D Lookup Table : Lookup_n-D  NumberOfTableDimensions=1  BreakpointsForDimension1=[-540 0 540]  Table=[-40 0 40]  InternalRulePriority=Speed  RndMeth=Simplest
  Saturation : Saturate  UpperLimit=40  LowerLimit=-40
  Scope1 : Scope  NumInputPorts=3
      settings: ActiveDisplayYMinimum=-1  ActiveDisplayYMaximum=1  DataLoggingVariableName=ScopeData19
  Str : Outport
  wires:
  Saturation/1 -> Str/1, Scope1/1
  1-D Lookup Table/1 -> Scope1/2, Saturation/1
  [SteerDM] -> 1-D Lookup Table/1, Scope1/3

== system SDV_HIL/HIL/Driver/Logitech G29 ==
  Add : Sum
  Add1 : Sum
  Constant : Constant  Value=50
  Constant1 : Constant  Value=8
  Demux : Demux
  Display : Display  Commented=on
  Display{2,4..6} (4 alike) : Display
  Display3 : Display  Commented=on
  Gain3 : Gain  Gain=-8
  Gain4 : Gain  Gain=-50
  Gain5 : Gain  Gain=40
  MATLAB Function : MATLAB Function  TreatAsAtomicUnit=on
  Selector : Selector  InputPortWidth=25  IndexOptions=Index vector (dialog)  Indices=[1]  OutputSizes=1
  Simulation 3D Joystick : sl3dlib/Simulation 3D/Hardware Interface/Simulation 3D Joystick  joyid=1  adjustports=on  forcefeed=off
  Terminator : Terminator
  Terminator2 : Terminator
  tag scope: BrakePXN=global, SteerPXN=global, ThrottlePXN=global
  wires:
  ? -> Terminator/1
  MATLAB Function/1(state) -> Display4/1
  Selector/1 -> MATLAB Function/1(btn)
  Gain5/1 -> [SteerPXN], Display2/1
  Add1/1 -> Display6/1, [BrakePXN]
  Constant1/1 -> Add1/2
  Gain3/1 -> Add1/1
  Demux/3 -> Gain3/1
  Demux/2 -> Display3/1, Gain4/1
  Demux/1 -> Gain5/1
  Demux/4 -> Terminator2/1
  Simulation 3D Joystick/1 -> Demux/1, Display/1
  Gain4/1 -> Add/1
  Constant/1 -> Add/2
  Simulation 3D Joystick/2 -> Selector/1
  Add/1 -> Display5/1, [ThrottlePXN]

== system SDV_HIL/HIL/Driver/Sine with Dwell ==
  Gain : Gain  Gain=5
  Sine with Dwell : SignalEditorBlockLib/Signal Editor  FileName=SineWithDwell_shifted.mat  ActiveScenario=Scenario  ActiveSignal=Signal 1  IsBus=off  OutputBusObjectStr=Bus: BusObject  SampleTime=0  ZeroCross=off  OutputAfterFinalValue=Setting to zero  Unit=inherit  PreserveSignalName=on  ApplySigPropsToAllScenarios=on  ApplySigPropsToAllSignals=off  SignalPropertySource=Dialog parameters
  Str : Outport
  wires:
  Gain/1 -> Str/1
  Sine with Dwell/1 -> Gain/1

== system SDV_HIL/HIL/Driver/Subsystem ==
  In1 : Inport
  Str : Outport
  wires:
  In1/1 -> Str/1

== system SDV_HIL/HIL/Sensor/Steering System ==
  In1 : Inport
  Demux : Demux  Outputs=14
  Terminator{,1..7} (8 alike) : Terminator
  tag scope: Lat_Path=global, Lat_Targ=global, Lat_Veh=global, SteerDM=global, sideslip_L2=global, sideslip_R2=global
  wires:
  In1/1 -> Demux/1
  Demux/1 -> Terminator/1
  Demux/2 -> Terminator1/1
  Demux/3 -> Terminator2/1
  Demux/4 -> Terminator3/1
  Demux/5 -> Terminator4/1
  Demux/6 -> Terminator5/1
  Demux/7 -> [SteerDM]
  Demux/8 -> [Lat_Targ]
  Demux/9 -> [Lat_Veh]
  Demux/10 -> [Lat_Path]
  Demux/11 -> Terminator6/1
  Demux/12 -> Terminator7/1
  Demux/13 -> [sideslip_L2]
  Demux/14 -> [sideslip_R2]

== system SDV_HIL/HIL/Sensor/Torque Vectoring ==
  In1 : Inport
  Degrees to Radians : simulink_extras/Transformations/Degrees to Radians
  Degrees to Radians2 : simulink_extras/Transformations/Degrees to Radians
  Demux : Demux  Outputs=15
  Mux : Mux
  Mux1 : Mux
  Mux2 : Mux
  Scope{,2..5} (5 alike) : Scope  Commented=on
      Scope settings: TimeSpan=10  ActiveDisplayYMinimum=-0.018082463921750395  ActiveDisplayYMaximum=0.017846570793703453  DataLoggingVariableName=ScopeData21
      Scope2 settings: ActiveDisplayYMinimum=-1  ActiveDisplayYMaximum=1  DataLoggingVariableName=ScopeData23
      Scope3 settings: ActiveDisplayYMinimum=-106.0637202101492  ActiveDisplayYMaximum=78.0503751303972  DataLoggingVariableName=ScopeData24
      Scope4 settings: ActiveDisplayYMinimum=6542.1615610939225  ActiveDisplayYMaximum=6577.8874866083952  DataLoggingVariableName=ScopeData25
      Scope5 settings: TimeSpan=10  ActiveDisplayYMinimum=-11.664536557177181  ActiveDisplayYMaximum=101.92313834201745  DataLoggingVariableName=ScopeData61
  Scope1 : Scope  Commented=on  NumInputPorts=2
      settings: ActiveDisplayYMinimum=-15.76512014934719  ActiveDisplayYMaximum=98.336342875694754  DataLoggingVariableName=ScopeData22
  tag scope: AngWheel=global, Fy=global, Fz=global, Vx=global, Vy=global, yawrate=global
  wires:
  In1/1 -> Demux/1
  Demux/1 -> Scope5/1, [Vx]
  Demux/2 -> Scope2/1, [Vy]
  Demux/3 -> Degrees to Radians/1
  Demux/4 -> Mux2/1
  Demux/5 -> Mux2/2
  Demux/6 -> Mux2/3
  Demux/7 -> Mux2/4
  Demux/8 -> Mux1/1
  Demux/9 -> Mux1/2
  Demux/10 -> Mux1/3
  Demux/11 -> Mux1/4
  Demux/12 -> Mux/1
  Demux/13 -> Mux/2
  Demux/14 -> Mux/3
  Demux/15 -> Mux/4
  Degrees to Radians/1 -> Scope/1, [yawrate]
  Mux/1 -> Scope3/1, [Fy]
  Mux1/1 -> Scope4/1, [Fz]
  Mux2/1 -> Scope1/2, Degrees to Radians2/1
  Degrees to Radians2/1 -> Scope1/1, [AngWheel]

== system SDV_HIL/HIL/Sensor/Traction Control ==
  In1 : Inport
  Demux : Demux  Outputs=14
  Gain{,1..3} (4 alike) : Gain  Gain=2*pi/60
  Mux : Mux
  Mux1 : Mux
  Terminator : Terminator
  g > m/s^2 : Gain  Gain=9.80665
  tag scope: Fx=global, VxWheel=global, Vx_L1=global, Vx_L2=global, Vx_R1=global, Vx_R2=global, ax=global, w_L1=global, w_L2=global, w_R1=global, w_R2=global
  wires:
  In1/1 -> Demux/1
  Demux/2 -> [Vx_L1]
  Demux/3 -> [Vx_R1]
  Demux/4 -> [Vx_L2]
  Demux/5 -> [Vx_R2]
  Demux/1 -> Terminator/1  "Vx"
  Demux/6 -> Gain/1
  Demux/7 -> Gain1/1
  Demux/8 -> Gain2/1
  Demux/9 -> Gain3/1
  Gain/1 -> [w_L1]
  Gain1/1 -> [w_R1]
  Gain2/1 -> [w_L2]
  Gain3/1 -> [w_R2]
  Demux/10 -> g > m/s^2/1
  g > m/s^2/1 -> [ax]
  Demux/14 -> Mux/4  "Fx_R2"
  Demux/13 -> Mux/3  "Fx_L2"
  Demux/12 -> Mux/2  "Fx_R1"
  Demux/11 -> Mux/1  "Fx_L1"
  Mux/1 -> [Fx]
  [Vx_L1] -> Mux1/1
  [Vx_R1] -> Mux1/2
  [Vx_L2] -> Mux1/3
  [Vx_R2] -> Mux1/4
  Mux1/1 -> [VxWheel]

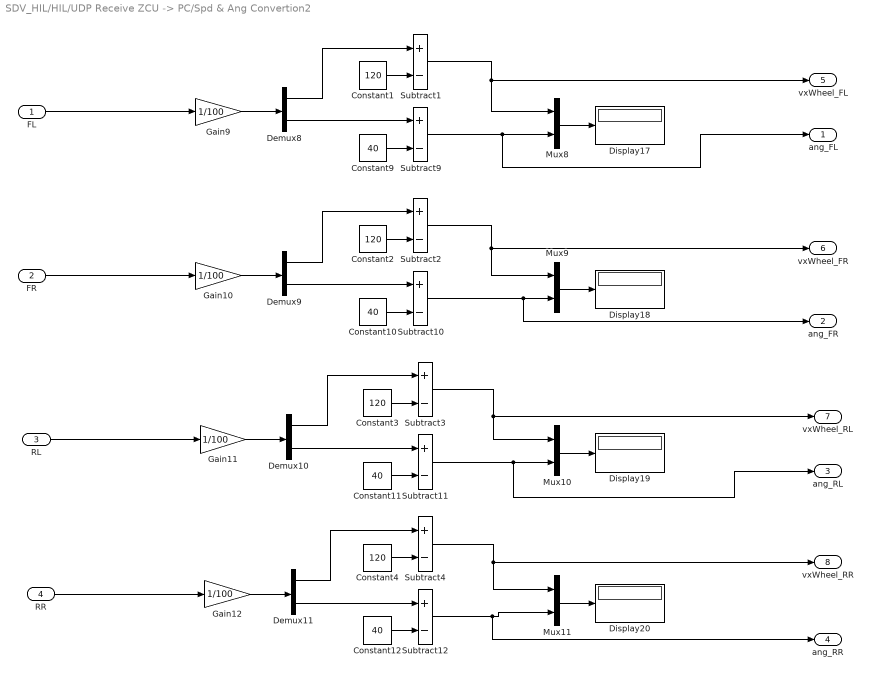
== system SDV_HIL/HIL/UDP Receive ZCU -> PC/Spd & Ang Convertion2 ==
  FL : Inport
  FR : Inport  Port=2
  RL : Inport  Port=3
  RR : Inport  Port=4
  Constant{1..4} (4 alike) : Constant  Value=120
  Constant{9..12} (4 alike) : Constant  Value=40
  Demux{8..11} (4 alike) : Demux  Outputs=2
  Display{17..20} (4 alike) : Display
  Gain{9..12} (4 alike) : Gain  Gain=1/100
  Mux{8..11} (4 alike) : Mux  Inputs=2
  Subtract{1..4,9..12} (8 alike) : Sum  Inputs=+-
  ang_FL : Outport
  ang_FR : Outport  Port=2
  ang_RL : Outport  Port=3
  ang_RR : Outport  Port=4
  vxWheel_FL : Outport  Port=5
  vxWheel_FR : Outport  Port=6
  vxWheel_RL : Outport  Port=7
  vxWheel_RR : Outport  Port=8
  wires:
  Gain12/1 -> Demux11/1
  Gain9/1 -> Demux8/1
  RR/1 -> Gain12/1
  FR/1 -> Gain10/1
  Gain10/1 -> Demux9/1
  Constant10/1 -> Subtract10/2
  Mux9/1 -> Display18/1
  Mux8/1 -> Display17/1
  FL/1 -> Gain9/1
  Mux10/1 -> Display19/1
  Constant12/1 -> Subtract12/2
  Mux11/1 -> Display20/1
  Gain11/1 -> Demux10/1
  Constant11/1 -> Subtract11/2
  Constant9/1 -> Subtract9/2
  RL/1 -> Gain11/1
  Subtract9/1 -> ang_FL/1, Mux8/2
  Subtract10/1 -> ang_FR/1, Mux9/2
  Subtract11/1 -> ang_RL/1, Mux10/2
  Subtract12/1 -> ang_RR/1, Mux11/2
  Constant1/1 -> Subtract1/2
  Demux8/1 -> Subtract1/1
  Subtract1/1 -> vxWheel_FL/1, Mux8/1
  Constant2/1 -> Subtract2/2
  Demux9/1 -> Subtract2/1
  Subtract2/1 -> vxWheel_FR/1, Mux9/1
  Constant3/1 -> Subtract3/2
  Demux10/1 -> Subtract3/1
  Subtract3/1 -> vxWheel_RL/1, Mux10/1
  Constant4/1 -> Subtract4/2
  Demux11/1 -> Subtract4/1
  Subtract4/1 -> vxWheel_RR/1, Mux11/1
  Demux8/2 -> Subtract9/1
  Demux9/2 -> Subtract10/1
  Demux10/2 -> Subtract11/1
  Demux11/2 -> Subtract12/1

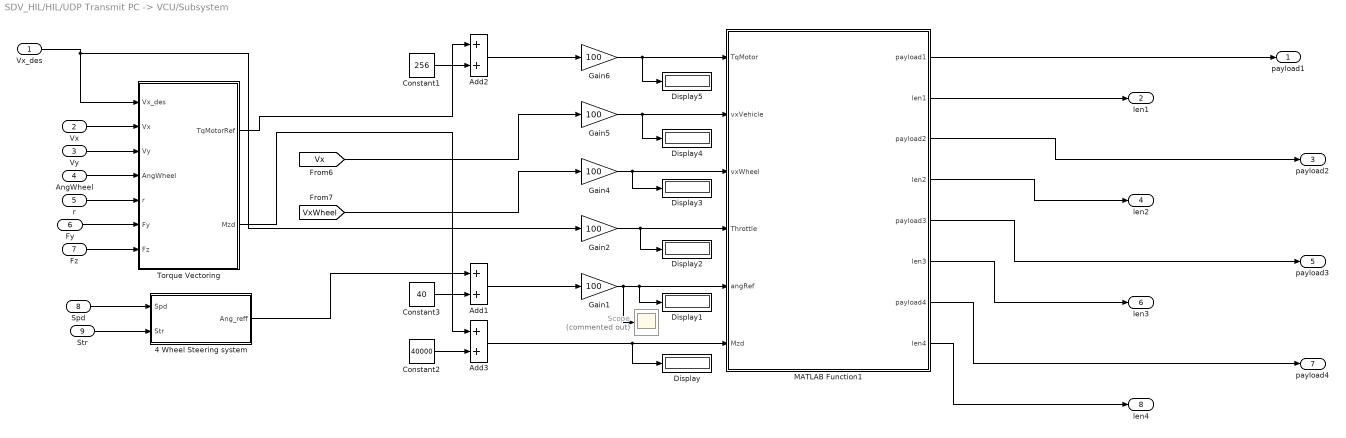
== system SDV_HIL/HIL/UDP Transmit PC -> VCU/Subsystem ==
  Vx_des : Inport
  Vx : Inport  Port=2
  Vy : Inport  Port=3
  AngWheel : Inport  Port=4
  r : Inport  Port=5
  Fy : Inport  Port=6
  Fz : Inport  Port=7
  Spd : Inport  Port=8
  Str : Inport  Port=9
  4 Wheel Steering system : Subsystem
  Add1 : Sum
  Add2 : Sum
  Add3 : Sum
  Constant1 : Constant  Value=256
  Constant2 : Constant  Value=40000
  Constant3 : Constant  Value=40
  Display{,1..5} (6 alike) : Display
  Gain{1..2,4..6} (5 alike) : Gain  Gain=100
  MATLAB Function1 : MATLAB Function  TreatAsAtomicUnit=on
  Scope : Scope  Commented=on
      settings: ActiveDisplayYMinimum=2651  ActiveDisplayYMaximum=5349  DataLoggingVariableName=ScopeData60
  Torque Vectoring : Subsystem
  payload1 : Outport
  len1 : Outport  Port=2
  payload2 : Outport  Port=3
  len2 : Outport  Port=4
  payload3 : Outport  Port=5
  len3 : Outport  Port=6
  payload4 : Outport  Port=7
  len4 : Outport  Port=8
  wires:
  Gain6/1 -> Display5/1, MATLAB Function1/1(TqMotor)
  Constant2/1 -> Add3/2
  Gain1/1 -> Display1/1, MATLAB Function1/5(angRef), Scope/1
  Gain2/1 -> Display2/1, MATLAB Function1/4(Throttle)
  AngWheel/1 -> Torque Vectoring/4(AngWheel)
  Fz/1 -> Torque Vectoring/7(Fz)
  4 Wheel Steering system/1(Ang_reff) -> Add1/1
  Vx_des/1 -> Torque Vectoring/1(Vx_des), Gain2/1
  Str/1 -> 4 Wheel Steering system/2(Str)
  MATLAB Function1/6(len3) -> len3/1
  r/1 -> Torque Vectoring/5(r)
  Gain5/1 -> Display4/1, MATLAB Function1/2(vxVehicle)
  Add3/1 -> Display/1, MATLAB Function1/6(Mzd)
  Torque Vectoring/1(TqMotorRef) -> Add2/1
  Torque Vectoring/2(Mzd) -> Add3/1
  Constant3/1 -> Add1/2
  Add2/1 -> Gain6/1
  Vy/1 -> Torque Vectoring/3(Vy)
  MATLAB Function1/3(payload2) -> payload2/1
  [VxWheel] -> Gain4/1
  Constant1/1 -> Add2/2
  Gain4/1 -> Display3/1, MATLAB Function1/3(vxWheel)
  Add1/1 -> Gain1/1
  MATLAB Function1/1(payload1) -> payload1/1
  MATLAB Function1/8(len4) -> len4/1
  [Vx] -> Gain5/1
  Vx/1 -> Torque Vectoring/2(Vx)
  Spd/1 -> 4 Wheel Steering system/1(Spd)
  MATLAB Function1/4(len2) -> len2/1
  Fy/1 -> Torque Vectoring/6(Fy)
  MATLAB Function1/7(payload4) -> payload4/1
  MATLAB Function1/5(payload3) -> payload3/1
  MATLAB Function1/2(len1) -> len1/1

== system SDV_HIL/HIL_VCU/Sensor/Steering System ==
  In1 : Inport
  Demux : Demux  Outputs=14
  Terminator{,1..7} (8 alike) : Terminator
  tag scope: Lat_Path=global, Lat_Targ=global, Lat_Veh=global, SteerDM=global, sideslip_L2=global, sideslip_R2=global
  wires:
  In1/1 -> Demux/1
  Demux/1 -> Terminator/1
  Demux/2 -> Terminator1/1
  Demux/3 -> Terminator2/1
  Demux/4 -> Terminator3/1
  Demux/5 -> Terminator4/1
  Demux/6 -> Terminator5/1
  Demux/7 -> [SteerDM]
  Demux/8 -> [Lat_Targ]
  Demux/9 -> [Lat_Veh]
  Demux/10 -> [Lat_Path]
  Demux/11 -> Terminator6/1
  Demux/12 -> Terminator7/1
  Demux/13 -> [sideslip_L2]
  Demux/14 -> [sideslip_R2]

== system SDV_HIL/HIL_VCU/Sensor/Torque Vectoring ==
  In1 : Inport
  Degrees to Radians : simulink_extras/Transformations/Degrees to Radians
  Degrees to Radians2 : simulink_extras/Transformations/Degrees to Radians
  Demux : Demux  Outputs=15
  Mux : Mux
  Mux1 : Mux
  Mux2 : Mux
  Scope{,2..5} (5 alike) : Scope  Commented=on
      Scope settings: TimeSpan=10  ActiveDisplayYMinimum=-0.018082463921750395  ActiveDisplayYMaximum=0.017846570793703453  DataLoggingVariableName=ScopeData21
      Scope2 settings: ActiveDisplayYMinimum=-1  ActiveDisplayYMaximum=1  DataLoggingVariableName=ScopeData23
      Scope3 settings: ActiveDisplayYMinimum=-106.0637202101492  ActiveDisplayYMaximum=78.0503751303972  DataLoggingVariableName=ScopeData24
      Scope4 settings: ActiveDisplayYMinimum=6542.1615610939225  ActiveDisplayYMaximum=6577.8874866083952  DataLoggingVariableName=ScopeData25
      Scope5 settings: TimeSpan=10  ActiveDisplayYMinimum=-11.664536557177181  ActiveDisplayYMaximum=101.92313834201745  DataLoggingVariableName=ScopeData61
  Scope1 : Scope  Commented=on  NumInputPorts=2
      settings: ActiveDisplayYMinimum=-15.76512014934719  ActiveDisplayYMaximum=98.336342875694754  DataLoggingVariableName=ScopeData22
  tag scope: AngWheel=global, Fy=global, Fz=global, Vx=global, Vy=global, yawrate=global
  wires:
  In1/1 -> Demux/1
  Demux/1 -> Scope5/1, [Vx]
  Demux/2 -> Scope2/1, [Vy]
  Demux/3 -> Degrees to Radians/1
  Demux/4 -> Mux2/1
  Demux/5 -> Mux2/2
  Demux/6 -> Mux2/3
  Demux/7 -> Mux2/4
  Demux/8 -> Mux1/1
  Demux/9 -> Mux1/2
  Demux/10 -> Mux1/3
  Demux/11 -> Mux1/4
  Demux/12 -> Mux/1
  Demux/13 -> Mux/2
  Demux/14 -> Mux/3
  Demux/15 -> Mux/4
  Degrees to Radians/1 -> Scope/1, [yawrate]
  Mux/1 -> Scope3/1, [Fy]
  Mux1/1 -> Scope4/1, [Fz]
  Mux2/1 -> Scope1/2, Degrees to Radians2/1
  Degrees to Radians2/1 -> Scope1/1, [AngWheel]

== system SDV_HIL/HIL_VCU/Sensor/Traction Control ==
  In1 : Inport
  Demux : Demux  Outputs=14
  Gain{,1..3} (4 alike) : Gain  Gain=2*pi/60
  Mux : Mux
  Mux1 : Mux
  Terminator : Terminator
  g > m/s^2 : Gain  Gain=9.80665
  tag scope: Fx=global, VxWheel=global, Vx_L1=global, Vx_L2=global, Vx_R1=global, Vx_R2=global, ax=global, w_L1=global, w_L2=global, w_R1=global, w_R2=global
  wires:
  In1/1 -> Demux/1
  Demux/2 -> [Vx_L1]
  Demux/3 -> [Vx_R1]
  Demux/4 -> [Vx_L2]
  Demux/5 -> [Vx_R2]
  Demux/1 -> Terminator/1  "Vx"
  Demux/6 -> Gain/1
  Demux/7 -> Gain1/1
  Demux/8 -> Gain2/1
  Demux/9 -> Gain3/1
  Gain/1 -> [w_L1]
  Gain1/1 -> [w_R1]
  Gain2/1 -> [w_L2]
  Gain3/1 -> [w_R2]
  Demux/10 -> g > m/s^2/1
  g > m/s^2/1 -> [ax]
  Demux/14 -> Mux/4  "Fx_R2"
  Demux/13 -> Mux/3  "Fx_L2"
  Demux/12 -> Mux/2  "Fx_R1"
  Demux/11 -> Mux/1  "Fx_L1"
  Mux/1 -> [Fx]
  [Vx_L1] -> Mux1/1
  [Vx_R1] -> Mux1/2
  [Vx_L2] -> Mux1/3
  [Vx_R2] -> Mux1/4
  Mux1/1 -> [VxWheel]

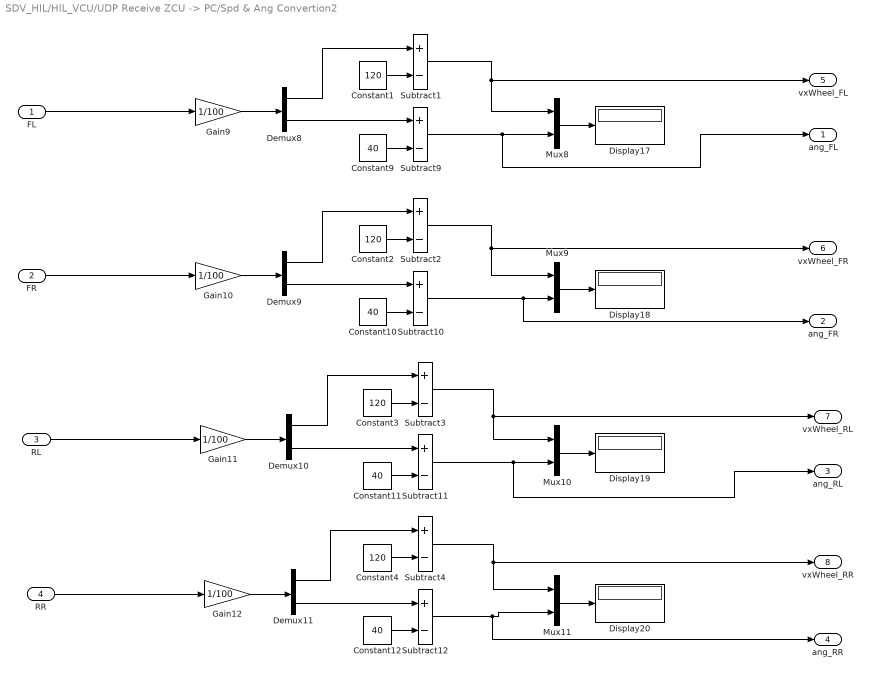
== system SDV_HIL/HIL_VCU/UDP Receive ZCU -> PC/Spd & Ang Convertion2 ==
  FL : Inport
  FR : Inport  Port=2
  RL : Inport  Port=3
  RR : Inport  Port=4
  Constant{1..4} (4 alike) : Constant  Value=120
  Constant{9..12} (4 alike) : Constant  Value=40
  Demux{8..11} (4 alike) : Demux  Outputs=2
  Display{17..20} (4 alike) : Display
  Gain{9..12} (4 alike) : Gain  Gain=1/100
  Mux{8..11} (4 alike) : Mux  Inputs=2
  Subtract{1..4,9..12} (8 alike) : Sum  Inputs=+-
  ang_FL : Outport
  ang_FR : Outport  Port=2
  ang_RL : Outport  Port=3
  ang_RR : Outport  Port=4
  vxWheel_FL : Outport  Port=5
  vxWheel_FR : Outport  Port=6
  vxWheel_RL : Outport  Port=7
  vxWheel_RR : Outport  Port=8
  wires:
  Gain12/1 -> Demux11/1
  Gain9/1 -> Demux8/1
  RR/1 -> Gain12/1
  FR/1 -> Gain10/1
  Gain10/1 -> Demux9/1
  Constant10/1 -> Subtract10/2
  Mux9/1 -> Display18/1
  Mux8/1 -> Display17/1
  FL/1 -> Gain9/1
  Mux10/1 -> Display19/1
  Constant12/1 -> Subtract12/2
  Mux11/1 -> Display20/1
  Gain11/1 -> Demux10/1
  Constant11/1 -> Subtract11/2
  Constant9/1 -> Subtract9/2
  RL/1 -> Gain11/1
  Subtract9/1 -> ang_FL/1, Mux8/2
  Subtract10/1 -> ang_FR/1, Mux9/2
  Subtract11/1 -> ang_RL/1, Mux10/2
  Subtract12/1 -> ang_RR/1, Mux11/2
  Constant1/1 -> Subtract1/2
  Demux8/1 -> Subtract1/1
  Subtract1/1 -> vxWheel_FL/1, Mux8/1
  Constant2/1 -> Subtract2/2
  Demux9/1 -> Subtract2/1
  Subtract2/1 -> vxWheel_FR/1, Mux9/1
  Constant3/1 -> Subtract3/2
  Demux10/1 -> Subtract3/1
  Subtract3/1 -> vxWheel_RL/1, Mux10/1
  Constant4/1 -> Subtract4/2
  Demux11/1 -> Subtract4/1
  Subtract4/1 -> vxWheel_RR/1, Mux11/1
  Demux8/2 -> Subtract9/1
  Demux9/2 -> Subtract10/1
  Demux10/2 -> Subtract11/1
  Demux11/2 -> Subtract12/1
